simulink model "PI_Laengsregler"  (R2019b)
settings: Solver=VariableStepAuto  StartTime=0.0  StopTime=20  MaxStep=0.01  RelTol=1e-3
libraries: simulink x1

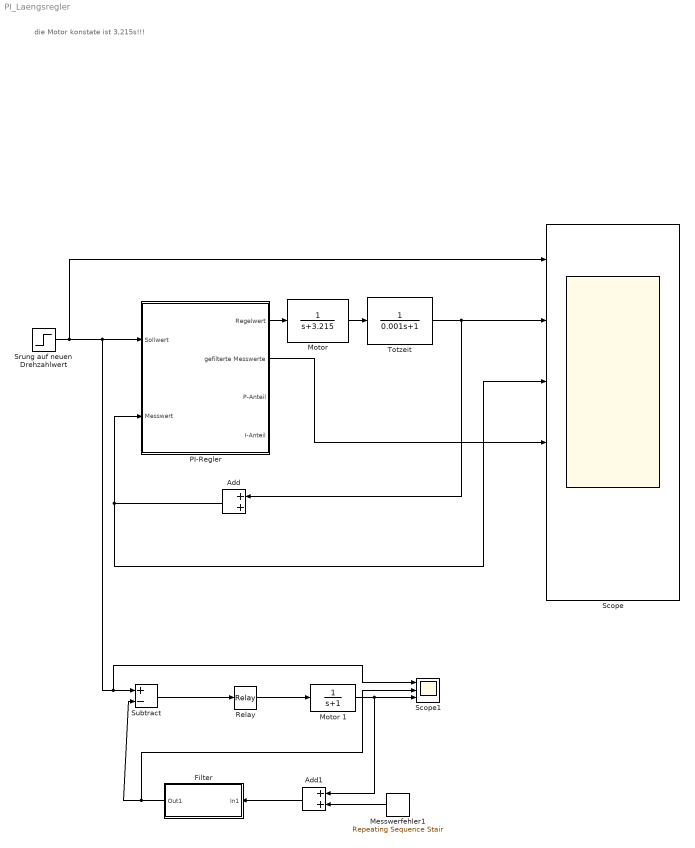
== system PI_Laengsregler ==
  note: die Motor konstate ist 3,215s!!!
  Add : Sum
  Add1 : Sum
  Filter : Subsystem
  Messwerfehler1 : simulink/Sources/Repeating Sequence Stair  OutValues="[0.3 0.1 -0.4  0.1 -0.2 0.1].'"  tsamp=-1  OutMin=[]  OutMax=[]  OutDataTypeStr=double  OutputDataTypeScalingMode=double  OutDataType=fixdt(0,8)  ConRadixGroup=Best Precision: Vector-wise  OutScaling=2^-12
  "Motor " : TransferFcn  Denominator=[1 3.215]
  Motor 1 : TransferFcn  Denominator=[1 1]
  PI-Regler : Subsystem
  Relay : Relay  OnSwitchValue=0.3  OffSwitchValue=-0.3  OnOutputValue=10
  Scope : Scope  NumInputPorts=6
  Scope1 : Scope  NumInputPorts=3
  Srung auf neuen Drehzahlwert : Step  SampleTime=0
  Subtract : Sum  Inputs=+-
  "Totzeit " : TransferFcn  Denominator=[0.001 1]
  wires:
  PI-Regler/1(Regelwert) -> "Motor "/1
  Srung auf neuen Drehzahlwert/1 -> Scope/1, Scope1/1, Subtract/1, PI-Regler/1(Sollwert)
  Add/1 -> PI-Regler/2(Messwert), Scope/3
  "Motor "/1 -> "Totzeit "/1
  PI-Regler/2(gefilterte Messwerte) -> Scope/4
  Subtract/1 -> Relay/1
  Relay/1 -> Motor 1/1
  Motor 1/1 -> Scope1/3, Add1/1
  Messwerfehler1/1 -> Add1/2
  Add1/1 -> Filter/1(In1)
  Filter/1(Out1) -> Scope1/2, Subtract/2
  "Totzeit "/1 -> Add/1, Scope/2

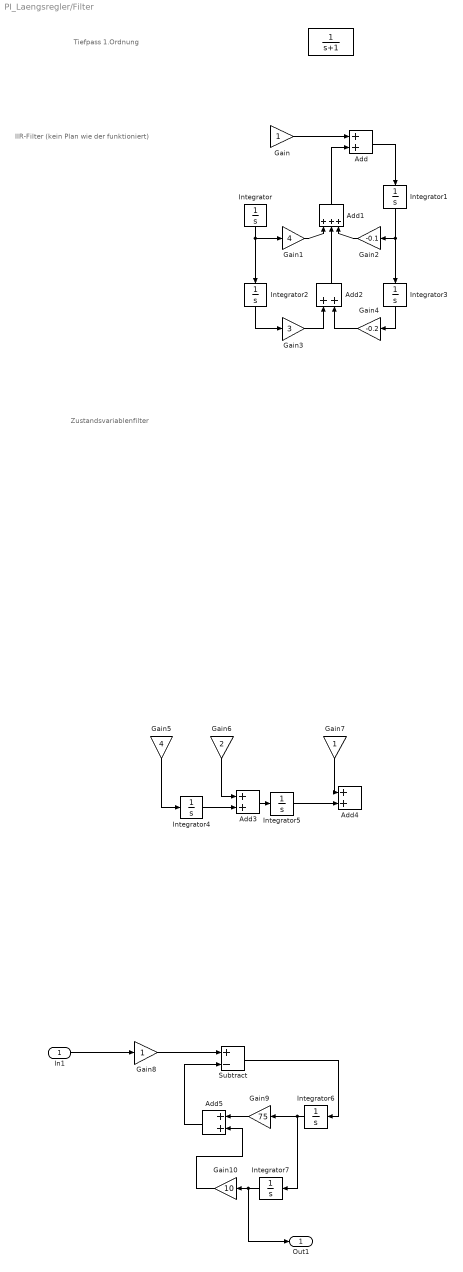
== system PI_Laengsregler/Filter ==
  note: Zustandsvariablenfilter
  note: IIR-Filter (kein Plan wie der funktioniert)
  note: Tiefpass 1.Ordnung
  In1 : Inport
  " " : TransferFcn  Denominator=[1 1]
  Add{,2..5} (5 alike) : Sum
  Add1 : Sum  Inputs=+++
  Gain : Gain
  Gain1 : Gain  Gain=4
  Gain10 : Gain  Gain=10
  Gain2 : Gain  Gain=-0.1
  Gain3 : Gain  Gain=3
  Gain4 : Gain  Gain=-0.2
  Gain5 : Gain  Gain=4
  Gain6 : Gain  Gain=2
  Gain7 : Gain
  Gain8 : Gain
  Gain9 : Gain  Gain=75
  Integrator{,1..7} (8 alike) : Integrator
  Subtract : Sum  Inputs=+-
  Out1 : Outport
  wires:
  Gain/1 -> Add/1
  Add/1 -> Integrator1/1
  Gain1/1 -> Add1/1
  Add1/1 -> Add/2
  Gain2/1 -> Add1/3
  Gain4/1 -> Add2/2
  Integrator3/1 -> Gain4/1
  Integrator2/1 -> Gain3/1
  Gain3/1 -> Add2/1
  Integrator1/1 -> Integrator3/1, Gain2/1
  Integrator/1 -> Integrator2/1, Gain1/1
  Add2/1 -> Add1/2
  Gain5/1 -> Integrator4/1
  Integrator4/1 -> Add3/2
  Gain6/1 -> Add3/1
  Add3/1 -> Integrator5/1
  Integrator5/1 -> Add4/2
  Gain7/1 -> Add4/1
  Gain8/1 -> Subtract/1
  Integrator6/1 -> Gain9/1, Integrator7/1
  Subtract/1 -> Integrator6/1
  Add5/1 -> Subtract/2
  Gain9/1 -> Add5/1
  Integrator7/1 -> Out1/1, Gain10/1
  Gain10/1 -> Add5/2
  In1/1 -> Gain8/1

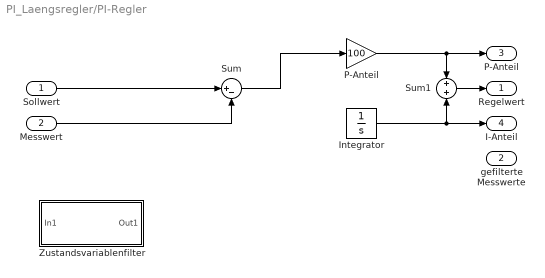
== system PI_Laengsregler/PI-Regler ==
  Sollwert : Inport
  Messwert : Inport  Port=2
  Integrator : Integrator
  "P-Anteil " : Gain  Gain=100
  Sum : Sum  Inputs=|+-
  Sum1 : Sum  Inputs=+|+
  Zustandsvariablenfilter : Subsystem
  Regelwert : Outport  VectorParamsAs1DForOutWhenUnconnected=off
  gefilterte Messwerte : Outport  Port=2
  P-Anteil : Outport  Port=3
  I-Anteil : Outport  Port=4
  wires:
  Sum/1 -> "P-Anteil "/1
  Integrator/1 -> I-Anteil/1, Sum1/2
  "P-Anteil "/1 -> Sum1/1, P-Anteil/1
  Sum1/1 -> Regelwert/1
  Sollwert/1 -> Sum/1
  Messwert/1 -> Sum/2

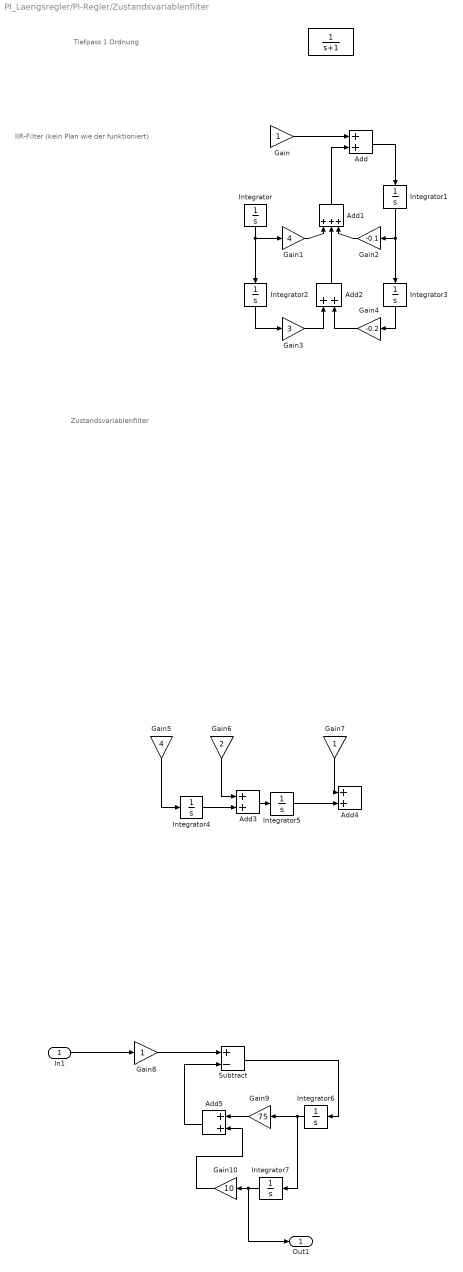
== system PI_Laengsregler/PI-Regler/Zustandsvariablenfilter ==
  note: Zustandsvariablenfilter
  note: IIR-Filter (kein Plan wie der funktioniert)
  note: Tiefpass 1.Ordnung
  In1 : Inport
  " " : TransferFcn  Denominator=[1 1]
  Add{,2..5} (5 alike) : Sum
  Add1 : Sum  Inputs=+++
  Gain : Gain
  Gain1 : Gain  Gain=4
  Gain10 : Gain  Gain=10
  Gain2 : Gain  Gain=-0.1
  Gain3 : Gain  Gain=3
  Gain4 : Gain  Gain=-0.2
  Gain5 : Gain  Gain=4
  Gain6 : Gain  Gain=2
  Gain7 : Gain
  Gain8 : Gain
  Gain9 : Gain  Gain=75
  Integrator{,1..7} (8 alike) : Integrator
  Subtract : Sum  Inputs=+-
  Out1 : Outport
  wires:
  Gain/1 -> Add/1
  Add/1 -> Integrator1/1
  Gain1/1 -> Add1/1
  Add1/1 -> Add/2
  Gain2/1 -> Add1/3
  Gain4/1 -> Add2/2
  Integrator3/1 -> Gain4/1
  Integrator2/1 -> Gain3/1
  Gain3/1 -> Add2/1
  Integrator1/1 -> Integrator3/1, Gain2/1
  Integrator/1 -> Integrator2/1, Gain1/1
  Add2/1 -> Add1/2
  Gain5/1 -> Integrator4/1
  Integrator4/1 -> Add3/2
  Gain6/1 -> Add3/1
  Add3/1 -> Integrator5/1
  Integrator5/1 -> Add4/2
  Gain7/1 -> Add4/1
  Gain8/1 -> Subtract/1
  Integrator6/1 -> Gain9/1, Integrator7/1
  Subtract/1 -> Integrator6/1
  Add5/1 -> Subtract/2
  Gain9/1 -> Add5/1
  Integrator7/1 -> Out1/1, Gain10/1
  Gain10/1 -> Add5/2
  In1/1 -> Gain8/1
